simulink model "optimizationtest"  (R2021a)
settings: Solver=VariableStepAuto  StartTime=0.0  StopTime=1.0  RelTol=1e-3
settings Model: Creator=alinjardan  LastModifiedBy=alinjardan

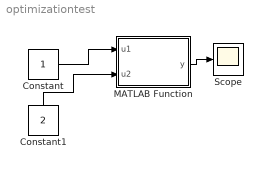
== system optimizationtest ==
  Constant : Constant
  Constant1 : Constant  Value=2
  MATLAB Function : MATLAB Function  TreatAsAtomicUnit=on
  Scope : Scope
  wires:
  Constant/1 -> MATLAB Function/1(u1)
  MATLAB Function/1(y) -> Scope/1
  Constant1/1 -> MATLAB Function/2(u2)

== matlab function optimizationtest/MATLAB Function ==
  data: u1 input; y output; u2 input
function y = fcn(u1,u2)
fun = @(x) x(1)^2+x(2)^2;
x0 = [u1;u2];
A = [1,2];
b = 2;
%options = optimoptions(@fmincon,'Algorithm','sqp','MaxIterations',1500);
options=optimoptions(@fmincon,'Algorithm','sqp');
x = fmincon(fun,x0,A,b,[],[],[],[],[],options);
y = x;
